simulink model "ex_model2"  (R2022b)
settings: configuration reference "Configuration" (kept outside this file)
libraries: ssreuselib x2, FixedLib x1
settings Model: Creator=amyyang  LastModifiedBy=amyyang
settings ConfigSetRef: SourceName=Configuration  SourceLocation=Base Workspace

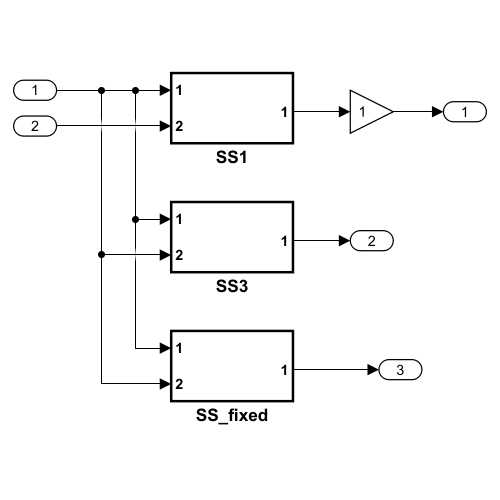
[thumbnail: Simulink's stored preview of the top-level diagram]
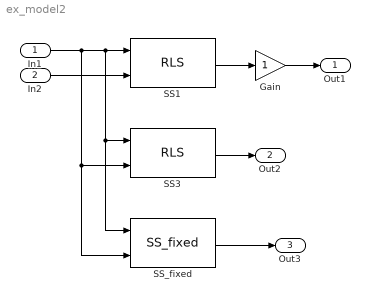
== system ex_model2 ==
  In1 : Inport
  In2 : Inport  Port=2
  Gain : Gain
  SS1 : ssreuselib/RLS  x=T1Break  y=T1Data
  SS3 : ssreuselib/RLS  x=T1Break  y=T1Data
  SS_fixed : FixedLib/SS_fixed  x=T1Break  y=T1Data
  Out1 : Outport
  Out2 : Outport  Port=2
  Out3 : Outport  Port=3
  wires:
  In2/1 -> SS1/2
  SS1/1 -> Gain/1
  SS3/1 -> Out2/1
  Gain/1 -> Out1/1
  SS_fixed/1 -> Out3/1
  In1/1 -> SS_fixed/2, SS3/2, SS_fixed/1, SS3/1, SS1/1
